simulink model "NetraAI_DigitalTwin_V4_District"  (Simulink 8.3)
settings: Solver=VariableStepDiscrete  StartTime=0.0  StopTime=28800  MaxStep=1  RelTol=1e-3
Description:
  | ANEYE / NetraAI Digital Twin V4 District Scenario. Target = 100000 screenings/year. Operating calendar, capture service, ophthalmology review and human-review times are explicit engineering assumptions. AI service time 8.67151 seconds is measured from one frozen reference case only. Balanced TRACE route mix is an engineering stress-test distribution and does not represent clinical prevalence.
settings Model: Creator=kaustav  LastModifiedBy=kaustav
settings DataIOCC: SignalLoggingSaveFormat=Dataset
settings DebuggingCC: UnderspecifiedInitializationDetection=Simplified  StateNameClashWarn=none
settings GRTTargetCC: CombineOutputUpdateFcns=on  GRTInterface=off

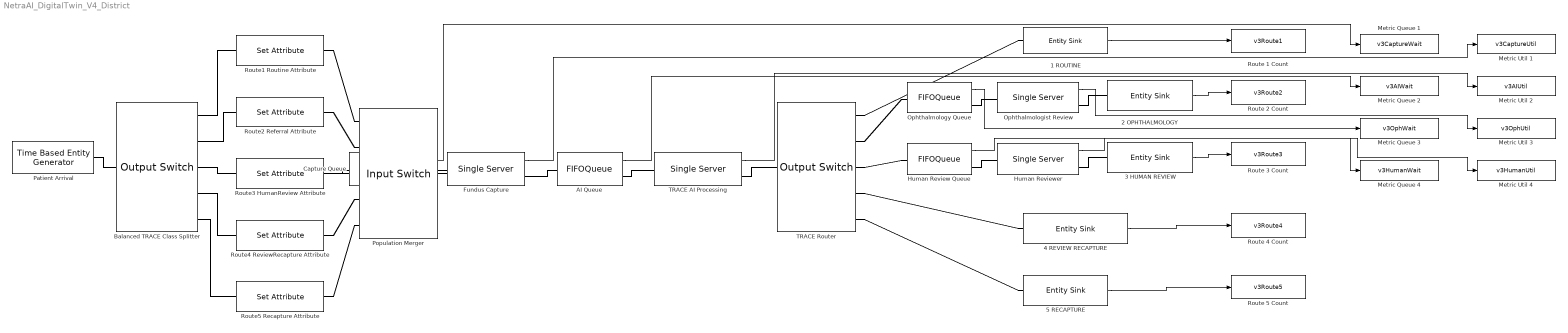
== system NetraAI_DigitalTwin_V4_District ==
  1 ROUTINE : EntitySink  StatNumberArrived=on
  2 OPHTHALMOLOGY : EntitySink  StatNumberArrived=on
  3 HUMAN REVIEW : EntitySink  StatNumberArrived=on
  4 REVIEW RECAPTURE : EntitySink  StatNumberArrived=on
  5 RECAPTURE : EntitySink  StatNumberArrived=on
  AI Queue : FIFOQueue  Capacity=1000  StatAverageWait=on
      settings: OutputPortMap=o2
  Balanced TRACE Class Splitter : OutputSwitch  NumberOutputPorts=5  SwitchingCriterion=Round robin
  Capture Queue : FIFOQueue  Capacity=1000  StatAverageWait=on
      settings: OutputPortMap=o2
  Fundus Capture : SingleServer  ServiceTime=120  StatUtilization=on
      settings: OutputPortMap=o5
  Human Review Queue : FIFOQueue  Capacity=1000  StatAverageWait=on
      settings: OutputPortMap=o2
  Human Reviewer : SingleServer  ServiceTime=45  StatUtilization=on
      settings: OutputPortMap=o5
  Metric Queue 1 : ToWorkspace  VariableName=v3CaptureWait  SampleTime=-1
  Metric Queue 2 : ToWorkspace  VariableName=v3AIWait  SampleTime=-1
  Metric Queue 3 : ToWorkspace  VariableName=v3OphWait  SampleTime=-1
  Metric Queue 4 : ToWorkspace  VariableName=v3HumanWait  SampleTime=-1
  Metric Util 1 : ToWorkspace  VariableName=v3CaptureUtil  SampleTime=-1
  Metric Util 2 : ToWorkspace  VariableName=v3AIUtil  SampleTime=-1
  Metric Util 3 : ToWorkspace  VariableName=v3OphUtil  SampleTime=-1
  Metric Util 4 : ToWorkspace  VariableName=v3HumanUtil  SampleTime=-1
  Ophthalmologist Review : SingleServer  ServiceTime=30  StatUtilization=on
      settings: OutputPortMap=o5
  Ophthalmology Queue : FIFOQueue  Capacity=1000  StatAverageWait=on
      settings: OutputPortMap=o2
  Patient Arrival : TimeBasedEntityGenerator  Period=86.4
  Population Merger : InputSwitch  NumberInputPorts=5
  Route 1 Count : ToWorkspace  VariableName=v3Route1  SampleTime=-1
  Route 2 Count : ToWorkspace  VariableName=v3Route2  SampleTime=-1
  Route 3 Count : ToWorkspace  VariableName=v3Route3  SampleTime=-1
  Route 4 Count : ToWorkspace  VariableName=v3Route4  SampleTime=-1
  Route 5 Count : ToWorkspace  VariableName=v3Route5  SampleTime=-1
  Route1 Routine Attribute : SetAttribute  AttributeName=routeCode  EvaluatedAttributeValue={ 1}
  Route2 Referral Attribute : SetAttribute  AttributeName=routeCode  AttributeValue=2  EvaluatedAttributeValue={ 2}
  Route3 HumanReview Attribute : SetAttribute  AttributeName=routeCode  AttributeValue=3  EvaluatedAttributeValue={ 3}
  Route4 ReviewRecapture Attribute : SetAttribute  AttributeName=routeCode  AttributeValue=4  EvaluatedAttributeValue={ 4}
  Route5 Recapture Attribute : SetAttribute  AttributeName=routeCode  AttributeValue=5  EvaluatedAttributeValue={ 5}
  TRACE AI Processing : SingleServer  ServiceTime=8.67151  StatUtilization=on
      settings: OutputPortMap=o5
  TRACE Router : OutputSwitch  NumberOutputPorts=5  SwitchingCriterion=From attribute  AttributeName=routeCode
  wires:
  1 ROUTINE/1 -> Route 1 Count/1
  2 OPHTHALMOLOGY/1 -> Route 2 Count/1
  3 HUMAN REVIEW/1 -> Route 3 Count/1
  4 REVIEW RECAPTURE/1 -> Route 4 Count/1
  5 RECAPTURE/1 -> Route 5 Count/1
  Capture Queue/1 -> Metric Queue 1/1
  AI Queue/1 -> Metric Queue 2/1
  Ophthalmology Queue/1 -> Metric Queue 3/1
  Human Review Queue/1 -> Metric Queue 4/1
  Fundus Capture/1 -> Metric Util 1/1
  TRACE AI Processing/1 -> Metric Util 2/1
  Ophthalmologist Review/1 -> Metric Util 3/1
  Human Reviewer/1 -> Metric Util 4/1
  connections:
  Route1 Routine Attribute/RConn1 -- Population Merger/LConn1
  Route2 Referral Attribute/RConn1 -- Population Merger/LConn2
  Route3 HumanReview Attribute/RConn1 -- Population Merger/LConn3
  Route4 ReviewRecapture Attribute/RConn1 -- Population Merger/LConn4
  Route5 Recapture Attribute/RConn1 -- Population Merger/LConn5
  Population Merger/RConn1 -- Capture Queue/LConn1
  Capture Queue/RConn1 -- Fundus Capture/LConn1
  Fundus Capture/RConn1 -- AI Queue/LConn1
  AI Queue/RConn1 -- TRACE AI Processing/LConn1
  TRACE AI Processing/RConn1 -- TRACE Router/LConn1
  TRACE Router/RConn1 -- 1 ROUTINE/LConn1
  TRACE Router/RConn2 -- Ophthalmology Queue/LConn1
  Ophthalmology Queue/RConn1 -- Ophthalmologist Review/LConn1
  Ophthalmologist Review/RConn1 -- 2 OPHTHALMOLOGY/LConn1
  TRACE Router/RConn3 -- Human Review Queue/LConn1
  Human Review Queue/RConn1 -- Human Reviewer/LConn1
  Human Reviewer/RConn1 -- 3 HUMAN REVIEW/LConn1
  TRACE Router/RConn4 -- 4 REVIEW RECAPTURE/LConn1
  TRACE Router/RConn5 -- 5 RECAPTURE/LConn1
  Patient Arrival/RConn1 -- Balanced TRACE Class Splitter/LConn1
  Balanced TRACE Class Splitter/RConn1 -- Route1 Routine Attribute/LConn1
  Balanced TRACE Class Splitter/RConn2 -- Route2 Referral Attribute/LConn1
  Balanced TRACE Class Splitter/RConn3 -- Route3 HumanReview Attribute/LConn1
  Balanced TRACE Class Splitter/RConn4 -- Route4 ReviewRecapture Attribute/LConn1
  Balanced TRACE Class Splitter/RConn5 -- Route5 Recapture Attribute/LConn1
